simulink model "Project_Simulink_1"  (R2023b)
settings: Solver=VariableStepAuto  StartTime=0.0  StopTime=100  RelTol=1e-3
settings Model: Creator=ricca  LastModifiedBy=Davide
settings SolverCC: AlgebraicLoopSolver=TrustRegion
settings DebuggingCC: UnconnectedInputMsg=warning  UnconnectedOutputMsg=warning  UnconnectedLineMsg=warning
settings ModelReferenceCC: EnableRefExpFcnMdlSchedulingChecks=on

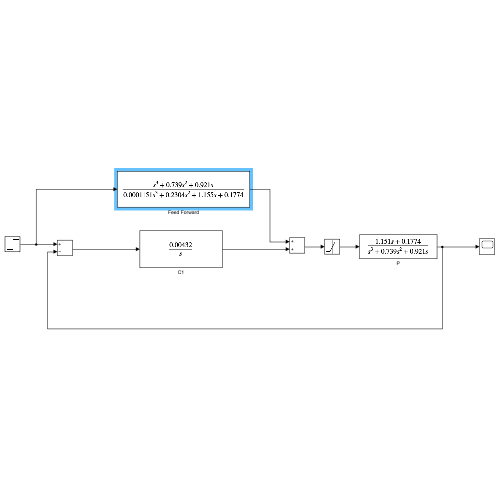
[thumbnail: Simulink's stored preview of the top-level diagram]
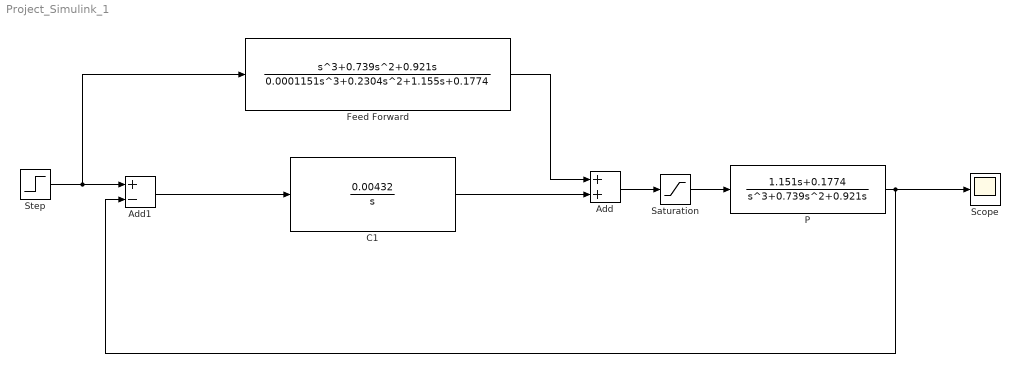
== system Project_Simulink_1 ==
  Add : Sum
  Add1 : Sum  Inputs=+-
  C1 : TransferFcn  Numerator=[0.00432]  Denominator=[1 0]
  Feed Forward : TransferFcn  Numerator=[1 0.739 0.921 0]  Denominator=[0.0001151 0.2304 1.155 0.1774]
  P : TransferFcn  Numerator=[1.151 0.1774]  Denominator=[1 0.739 0.921 0]
  Saturation : Saturate  UpperLimit=2  LowerLimit=-2
  Scope : Scope
  Step : Step  SampleTime=0
  wires:
  P/1 -> Scope/1, Add1/2
  Step/1 -> Feed Forward/1, Add1/1
  Add1/1 -> C1/1
  C1/1 -> Add/2
  Saturation/1 -> P/1
  Add/1 -> Saturation/1
  Feed Forward/1 -> Add/1
